simulink model "CruiseControl_LQR_Controller"  (R2026a)
settings: Solver=ode45  StopTime=120.0
settings Model: Creator=YASHRK  LastModifiedBy=YASHRK

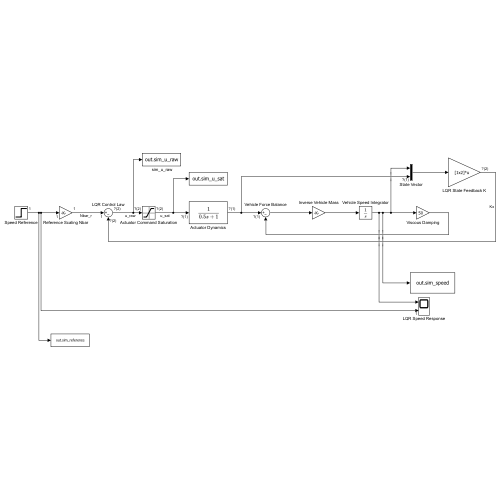
[thumbnail: Simulink's stored preview of the top-level diagram]
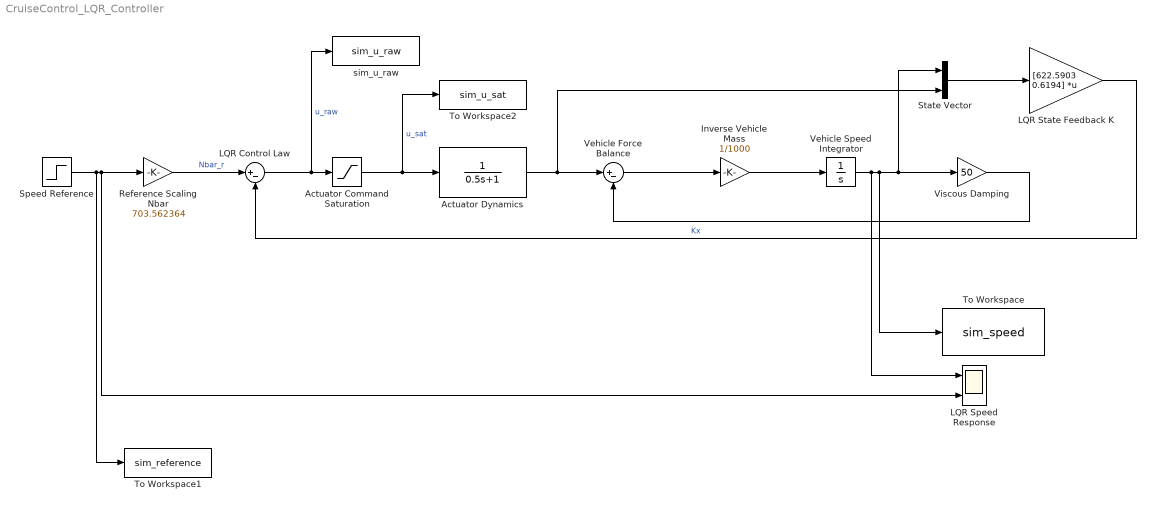
== system CruiseControl_LQR_Controller ==
  " sim_u_raw" : ToWorkspace  VariableName=sim_u_raw  SaveFormat=Timeseries  SampleTime=-1
  Actuator Command Saturation : Saturate  UpperLimit=700  LowerLimit=-700
  Actuator Dynamics : TransferFcn  Denominator=[0.5 1]
  Inverse Vehicle Mass : Gain  Gain=1/1000
  LQR Control Law : Sum  Inputs=|+-
  LQR Speed Response : Scope  NumInputPorts=2
  LQR State Feedback K : Gain  Gain=[622.5903 0.6194]  Multiplication=Matrix(K*u)
  Reference Scaling Nbar : Gain  Gain=703.562364
  Speed Reference : Step  Time=0  SampleTime=0
  State Vector : Mux  Inputs=2
  To Workspace : ToWorkspace  VariableName=sim_speed  SaveFormat=Timeseries  SampleTime=-1
  To Workspace1 : ToWorkspace  VariableName=sim_reference  SaveFormat=Timeseries  SampleTime=-1
  To Workspace2 : ToWorkspace  VariableName=sim_u_sat  SaveFormat=Timeseries  SampleTime=-1
  Vehicle Force Balance : Sum  Inputs=|+-
  Vehicle Speed Integrator : Integrator
  Viscous Damping : Gain  Gain=50
  wires:
  Vehicle Force Balance/1 -> Inverse Vehicle Mass/1
  Inverse Vehicle Mass/1 -> Vehicle Speed Integrator/1
  Vehicle Speed Integrator/1 -> LQR Speed Response/1, To Workspace/1, State Vector/1, Viscous Damping/1
  Viscous Damping/1 -> Vehicle Force Balance/2
  Actuator Dynamics/1 -> State Vector/2, Vehicle Force Balance/1
  State Vector/1 -> LQR State Feedback K/1
  Speed Reference/1 -> To Workspace1/1, Reference Scaling Nbar/1, LQR Speed Response/2
  Reference Scaling Nbar/1 -> LQR Control Law/1  "Nbar_r"
  LQR State Feedback K/1 -> LQR Control Law/2  "Kx"
  LQR Control Law/1 -> Actuator Command Saturation/1, " sim_u_raw"/1  "u_raw"
  Actuator Command Saturation/1 -> To Workspace2/1, Actuator Dynamics/1  "u_sat"
